simulink library "governor_lib"  (R2022b)
settings: Solver=VariableStepAuto  StartTime=0.0  StopTime=10.0  RelTol=1e-3
undefined symbols (not defined in the file): BM_STATUSES, DI_STATUSES, MI_STATUSES
settings Model: Creator=dr_pa  LastModifiedBy=dr_pa

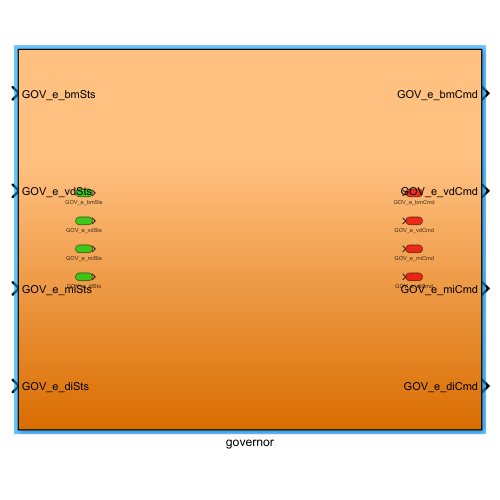
[thumbnail: Simulink's stored preview of the top-level diagram]
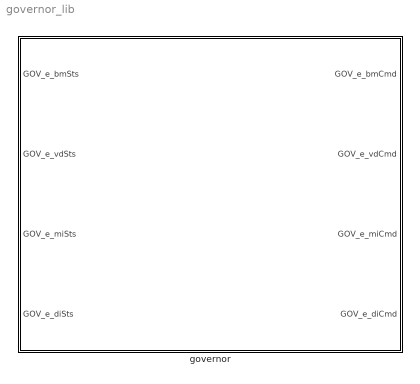
== system governor_lib ==
  governor : Subsystem

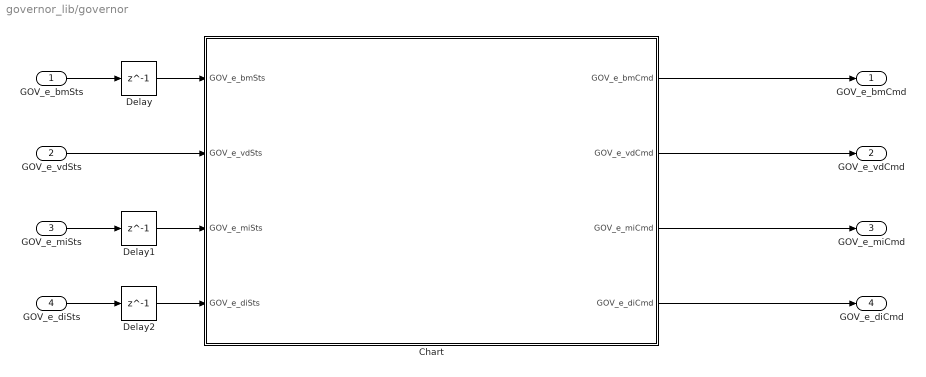
== system governor_lib/governor ==
  GOV_e_bmSts : Inport
  GOV_e_vdSts : Inport  Port=2
  GOV_e_miSts : Inport  Port=3
  GOV_e_diSts : Inport  Port=4
  Chart : Stateflow chart  TreatAsAtomicUnit=on
  Delay : Delay  DelayLength=1  InitialCondition=BM_STATUSES.BM_UNKNOWN
  Delay1 : Delay  DelayLength=1  InitialCondition=MI_STATUSES.UNKNOWN
  Delay2 : Delay  DelayLength=1  InitialCondition=DI_STATUSES.DI_UNKNOWN
  GOV_e_bmCmd : Outport
  GOV_e_vdCmd : Outport  Port=2
  GOV_e_miCmd : Outport  Port=3
  GOV_e_diCmd : Outport  Port=4
  wires:
  GOV_e_bmSts/1 -> Delay/1
  GOV_e_vdSts/1 -> Chart/2(GOV_e_vdSts)
  GOV_e_diSts/1 -> Delay2/1
  Chart/1(GOV_e_bmCmd) -> GOV_e_bmCmd/1
  Chart/2(GOV_e_vdCmd) -> GOV_e_vdCmd/1
  Chart/3(GOV_e_miCmd) -> GOV_e_miCmd/1
  Chart/4(GOV_e_diCmd) -> GOV_e_diCmd/1
  GOV_e_miSts/1 -> Delay1/1
  Delay/1 -> Chart/1(GOV_e_bmSts)
  Delay1/1 -> Chart/3(GOV_e_miSts)
  Delay2/1 -> Chart/4(GOV_e_diSts)

== stateflow chart governor_lib/governor/Chart ==
  state Initialize_outputs
    en:
    GOV_e_bmCmd = 0;
    GOV_e_vdCmd = 0;
    GOV_e_miCmd = MI_CMD.CMD_INIT;
    GOV_e_diCmd = DI_CMD.DI_CMD_INIT;
    motorStartCount = 0;
  state STARTUP
    state HV_startup
      en:
    state Command_motor_startup
      en:
      GOV_e_miCmd = MI_CMD.CMD_STARTUP;
      motorStartCount = motorStartCount+1;
    state Send_ReadyToDrive
      en:
      GOV_e_diCmd = DI_CMD.READY_TO_DRIVE;
    (default) -> HV_startup
    HV_startup -> Command_motor_startup : [GOV_e_bmSts == BM_STATUSES.BM_RUNNING]
    Command_motor_startup -> (junction 95) : [GOV_e_miSts == ...
        | MI_STATUSES.RUNNING]
    (junction 95) -> Send_ReadyToDrive : [GOV_e_diSts == ...
        | DI_STATUSES.DRV_START_REQ]
  state STARTUP_ERROR
    state HV_startup_error
      en:
    state Err_reset
      during:
      GOV_e_miCmd=...
      MI_CMD.CMD_SHUTDOWN;
      GOV_e_miCmd=...
      MI_CMD.ERR_RESET;
    state Motor_faulted
      en:
      % tell other motor to shutdown
      % if still running
      GOV_e_miCmd=...
      MI_CMD.CMD_SHUTDOWN;
    state DriverInterface_Error
      en:
    (junction 88) -> Err_reset [order 2]
    (junction 88) -> Motor_faulted [order 1] : [motorStartCount >= 5]
  state RUNNING_ERROR
    state HV_run_error
      en:
      GOV_e_diCmd = ...
      DI_CMD.SYSTEM_ERROR;
    state Motor_run_error
      en:
      GOV_e_diCmd = ...
      DI_CMD.SYSTEM_ERROR;
  state RUNNING
    en:
  (default) -> Initialize_outputs
  Initialize_outputs -> HV_startup
  STARTUP -> HV_startup_error [order 1] : [GOV_e_bmSts == ...
      | BM_STATUSES.ERR_STARTUP]
  Err_reset -> STARTUP : [GOV_e_miSts ==...
      |  MI_STATUSES.OFF]
  STARTUP -> (junction 88) [order 3] : [GOV_e_miSts == ...
      | MI_STATUSES.ERROR]
  STARTUP -> DriverInterface_Error [order 2] : [GOV_e_diSts ==...
      | DI_STATUSES.DI_ERROR]
  Send_ReadyToDrive -> RUNNING : [GOV_e_diSts == ...
      | DI_STATUSES.DI_RUNNING]
  RUNNING -> HV_run_error [order 1] : [GOV_e_bmSts == ...
      | BM_STATUSES.ERR_STARTUP]
  RUNNING -> Motor_run_error [order 2] : [GOV_e_miSts == ...
      | MI_STATUSES.ERROR]
  data: GOV_e_bmSts input; GOV_e_vdSts input; GOV_e_miSts input; GOV_e_diSts input; GOV_e_bmCmd output uint8 size=1; GOV_e_vdCmd output uint8 size=1; GOV_e_miCmd output Enum: MI_CMD size=1; GOV_e_diCmd output Enum: DI_CMD size=1; motorStartCount local uint16
